simulink model "sfcndemo_atmos"  (Simulink 7.6)
settings: Solver=ode1  StartTime=0.0  StopTime=1200  RelTol=1e-3
libraries: simulink x1
Description:
  | Example of C calling Fortran - Atmospheric Properties
  | 
  | This is a simulation-only demonstration of how a Level-2 C-MEX S-function can be
  | used as a wrapper to call Fortran code for simulation purposes.  This is documented
  | in the "Writing S-functions" manual that is part of the SImulink documentation set.  This
  | demonstration does *not* provide support for integration of Fortran with Real-Time
  | Workshop code generation.
settings Model: RequirementInfo=9  Creator=The MathWorks Inc.  ExtModeAutoUpdateStatusClock=off  BufferReuse=off
settings OptimizationCC: BlockReduction=off  BooleanDataType=off  InlineParams=on  OptimizeBlockIOStorage=off  BufferReuse=off  ExpressionFolding=off  LocalBlockOutputs=off  InitFltsAndDblsToZero=on  BufferReusableBoundary=off
settings DebuggingCC: SaveWithParameterizedLinksMsg=none  SignalResolutionControl=TryResolveAllWithWarning  SolverPrmCheckMsg=none  MultiTaskDSMMsg=warning  MultiTaskCondExecSysMsg=none
settings HardwareCC: TargetUnknown=on
settings RTWCC: IncludeERTFirstTime=on
settings CodeAppCC: CustomSymbolStrFcn=$F$N$M
settings GRTTargetCC: TargetFcnLib=ansi_tfl_tmw.mat

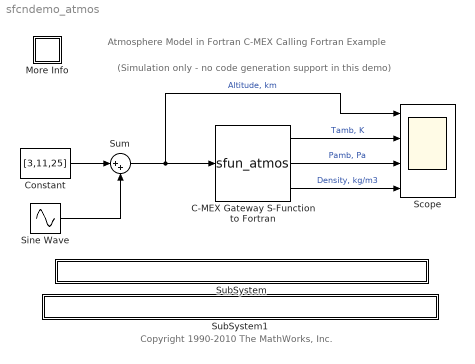
== system sfcndemo_atmos ==
  note: Atmosphere Model in Fortran
      | C-MEX Calling Fortran Example
  note: (Simulation only - no code generation support in this demo)
  note: Copyright 1990-2010 The MathWorks, Inc.
  C-MEX Gateway S-Function to Fortran : S-Function  FunctionName=sfun_atmos  Parameters=288.15,101325.0,0.0103  EnableBusSupport=off
  Constant : Constant  Value=[3,11,25]
  More Info : Subsystem
      mask Display: disp('?')
  Scope : Scope  NumInputPorts=4
      settings: TimeRange=1200  YMin=0~200~0~0  YMax=30~300~150000~0.015
  Sine Wave : Sin  Amplitude=3  Frequency=0.01  SampleTime=0
  SubSystem : Subsystem  mask{filename=sfun_atmos.c}
      mask init:
      | x=sfundemo_maskdisp;
      settings: AttributesFormatString=\n  OpenFcn=sfundemo_openfcn
      mask Display: disp(['gateway: ' x]);
  SubSystem1 : Subsystem  mask{filename=sfun_atmos_sub.F}
      mask init:
      | x=sfundemo_maskdisp;
      settings: AttributesFormatString=\n  OpenFcn=sfundemo_openfcn
      mask Display: disp(['Fortran: ' x]);
  Sum : Sum  Inputs=|++  SaturateOnIntegerOverflow=on  InputSameDT=on  OutDataTypeStr=Inherit: Same as first input
  wires:
  Constant/1 -> Sum/1
  Sine Wave/1 -> Sum/2
  Sum/1 -> C-MEX Gateway S-Function to Fortran/1, Scope/1  "Altitude, km"
  C-MEX Gateway S-Function to Fortran/1 -> Scope/2  "Tamb, K"
  C-MEX Gateway S-Function to Fortran/2 -> Scope/3  "Pamb, Pa"
  C-MEX Gateway S-Function to Fortran/3 -> Scope/4  "Density, kg/m3"

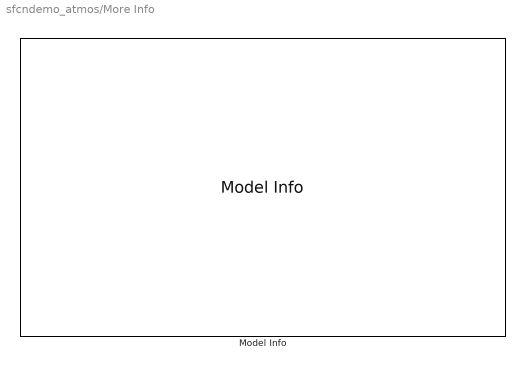
== system sfcndemo_atmos/More Info ==
  Model Info : simulink/Model-Wide Utilities/Model Info  InitialBlockCM=none  BlockCM=none  Frame=on  DisplayStringWithTags=|  HorizontalTextAlignment=Left  LeftAlignmentValue=0.02  SourceBlockDiagram=sfcndemo_atmos  TagMaxNumber=20
      | Model Description:
      | -------------------
      | 
      | %<Description>

== system sfcndemo_atmos/SubSystem ==

== system sfcndemo_atmos/SubSystem1 ==
